simulink model "problem2"  (R2020a)
settings: Solver=VariableStepAuto  StartTime=0.0  StopTime=100  FixedStep=0.6  MaxStep=0.2  RelTol=1e-3
values from neighbouring files (symbols this model uses):
  k1 = 80000    [bumpyroad.m]
  k2 = 500000    [bumpyroad.m]
  m1 = 2500    [bumpyroad.m]
  m2 = 320    [bumpyroad.m]
undefined symbols (not defined in the file or in its folder): b
settings Model: Creator=I3  LastModifiedBy=I3
settings SolverCC: AlgebraicLoopSolver=LineSearch
settings DataIOCC: ExternalInput=[t, stin]  LoadExternalInput=on  SaveFormat=Array

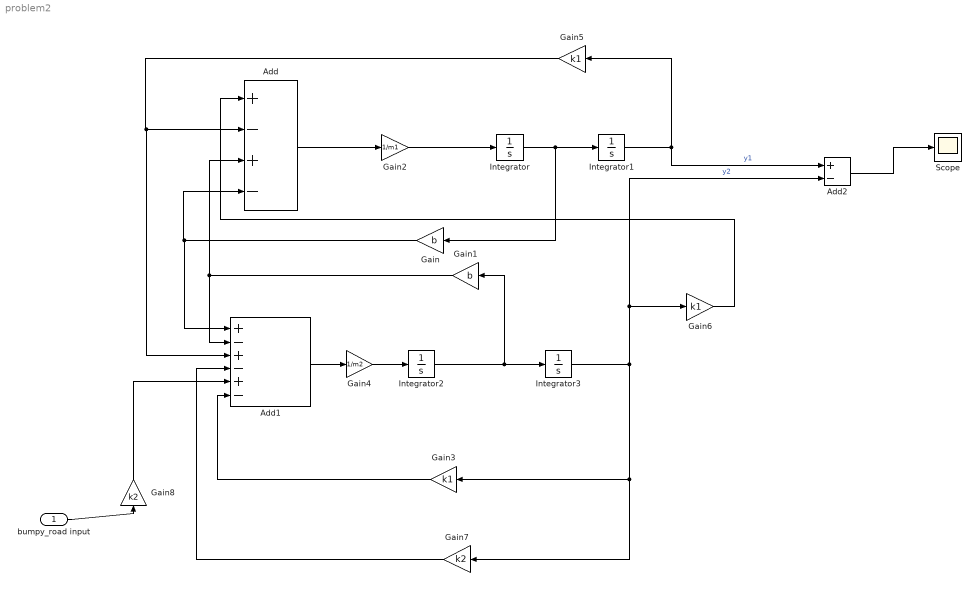
== system problem2 ==
  bumpy_road input : Inport
  Add : Sum  Inputs=+-+-
  Add1 : Sum  Inputs=+-+-+-
  Add2 : Sum  Inputs=+-
  Gain : Gain  Gain=b
  Gain1 : Gain  Gain=b
  Gain2 : Gain  Gain=1/m1
  Gain3 : Gain  Gain=k1
  Gain4 : Gain  Gain=1/m2
  Gain5 : Gain  Gain=k1
  Gain6 : Gain  Gain=k1
  Gain7 : Gain  Gain=k2
  Gain8 : Gain  Gain=k2
  Integrator{,1..3} (4 alike) : Integrator
  Scope : Scope
  wires:
  Integrator1/1 -> Add2/1, Gain5/1  "y1"
  Integrator2/1 -> Gain1/1, Integrator3/1
  Integrator/1 -> Gain/1, Integrator1/1
  Gain2/1 -> Integrator/1
  Add/1 -> Gain2/1
  Add1/1 -> Gain4/1
  Gain4/1 -> Integrator2/1
  Gain/1 -> Add1/1, Add/4
  Gain1/1 -> Add1/2, Add/3
  Gain5/1 -> Add1/3, Add/2
  Gain6/1 -> Add/1
  Gain3/1 -> Add1/6
  Gain7/1 -> Add1/4
  Gain8/1 -> Add1/5
  Integrator3/1 -> Gain7/1, Gain3/1, Add2/2, Gain6/1  "y2"
  Add2/1 -> Scope/1
  bumpy_road input/1 -> Gain8/1
